simulink model "lab8_3and4"  (R2018b)
settings: Solver=FixedStepDiscrete  StartTime=0.0  StopTime=1000000  FixedStep=1  RelTol=1e-3
libraries: hdlsllib x4, simulink x2
settings Model: Creator=mllax8  LastModifiedBy=mllax8

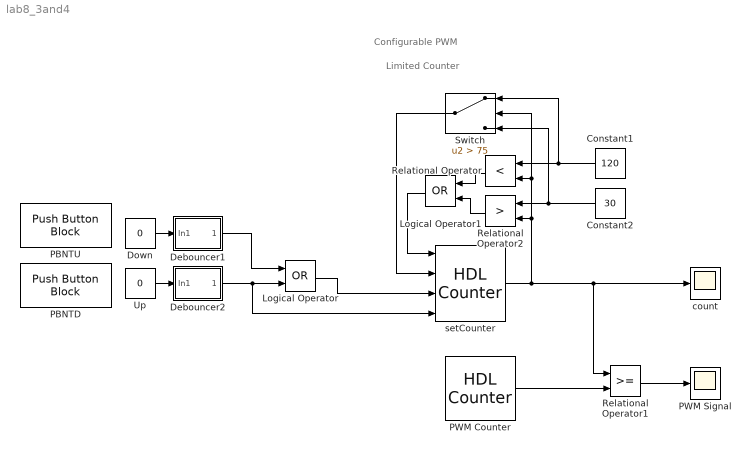
== system lab8_3and4 ==
  note: Configurable PWM
  note: Limited Counter
  Constant1 : Constant  Value=120  SampleTime=1
  Constant2 : Constant  Value=30  SampleTime=1
  Debouncer1 : Subsystem
  Debouncer2 : Subsystem
  Down : Constant  Value=0
  Logical Operator : Logic  Operator=OR  AllPortsSameDT=off  OutDataTypeStr=boolean
  Logical Operator1 : Logic  Operator=OR  AllPortsSameDT=off  OutDataTypeStr=boolean
  PBNTD : PushButtonBlock  WebBlockId=8
  PBNTU : PushButtonBlock  WebBlockId=9
  "PWM Counter " : hdlsllib/Sources/HDL Counter  CountType=Count limited  CountInit=0  CountStep=1  CountMax=1000  CountFromType=Initial value  CountFrom=0  CountResetPort=off  CountLoadPort=off  CountEnbPort=off  CountDirPort=off  CountDataType=Unsigned  CountWordLen=18  CountFracLen=0  CountSampTime=1
      settings: SourceProductBaseCode=HD
  PWM Signal : Scope
  Relational Operator : RelationalOperator  Operator=<  OutDataTypeStr=boolean  RndMeth=Simplest
  Relational Operator1 : RelationalOperator  OutDataTypeStr=boolean  RndMeth=Simplest
  Relational Operator2 : RelationalOperator  Operator=>  OutDataTypeStr=boolean  RndMeth=Simplest
  Switch : Switch  Criteria=u2 > Threshold  Threshold=75
  Up : Constant  Value=0
  count : Scope
  setCounter : hdlsllib/Sources/HDL Counter  CountType=Free running  CountInit=75  CountStep=6  CountMax=120  CountFromType=Initial value  CountFrom=75  CountResetPort=off  CountLoadPort=on  CountEnbPort=on  CountDirPort=on  CountDataType=Unsigned  CountWordLen=8  CountFracLen=0  CountSampTime=1
      settings: SourceProductBaseCode=HD
  wires:
  Down/1 -> Debouncer1/1(In1)
  Up/1 -> Debouncer2/1(In1)
  Debouncer1/1(Out1) -> Logical Operator/1
  Relational Operator1/1 -> PWM Signal/1
  Constant1/1 -> Switch/1, Relational Operator/1
  Constant2/1 -> Switch/3, Relational Operator2/1
  Logical Operator/1 -> setCounter/3
  Switch/1 -> setCounter/2
  Logical Operator1/1 -> setCounter/1
  setCounter/1 -> count/1, Relational Operator1/1, Switch/2, Relational Operator/2, Relational Operator2/2
  "PWM Counter "/1 -> Relational Operator1/2
  Relational Operator2/1 -> Logical Operator1/2
  Relational Operator/1 -> Logical Operator1/1
  Debouncer2/1(Out1) -> setCounter/4, Logical Operator/2

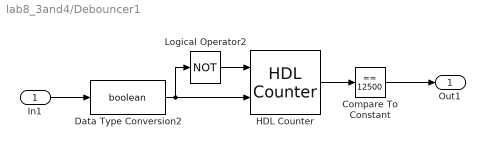
== system lab8_3and4/Debouncer1 ==
  In1 : Inport
  Compare To Constant : simulink/Logic and Bit Operations/Compare To Constant  relop===  const=12500  OutDataTypeStr=boolean
  Data Type Conversion2 : DataTypeConversion  OutDataTypeStr=boolean
  "HDL Counter " : hdlsllib/Sources/HDL Counter  CountType=Count limited  CountInit=0  CountStep=1  CountMax=50000  CountFromType=Initial value  CountFrom=0  CountResetPort=on  CountLoadPort=off  CountEnbPort=on  CountDirPort=off  CountDataType=Unsigned  CountWordLen=18  CountFracLen=0  CountSampTime=1
      settings: SourceProductBaseCode=HD
  Logical Operator2 : Logic  Operator=NOT  AllPortsSameDT=off  OutDataTypeStr=boolean
  Out1 : Outport
  wires:
  "HDL Counter "/1 -> Compare To Constant/1
  In1/1 -> Data Type Conversion2/1
  Logical Operator2/1 -> "HDL Counter "/1
  Compare To Constant/1 -> Out1/1
  Data Type Conversion2/1 -> "HDL Counter "/2, Logical Operator2/1

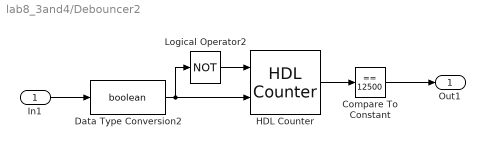
== system lab8_3and4/Debouncer2 ==
  In1 : Inport
  Compare To Constant : simulink/Logic and Bit Operations/Compare To Constant  relop===  const=12500  OutDataTypeStr=boolean
  Data Type Conversion2 : DataTypeConversion  OutDataTypeStr=boolean
  "HDL Counter " : hdlsllib/Sources/HDL Counter  CountType=Count limited  CountInit=0  CountStep=1  CountMax=50000  CountFromType=Initial value  CountFrom=0  CountResetPort=on  CountLoadPort=off  CountEnbPort=on  CountDirPort=off  CountDataType=Unsigned  CountWordLen=18  CountFracLen=0  CountSampTime=1
      settings: SourceProductBaseCode=HD
  Logical Operator2 : Logic  Operator=NOT  AllPortsSameDT=off  OutDataTypeStr=boolean
  Out1 : Outport
  wires:
  "HDL Counter "/1 -> Compare To Constant/1
  In1/1 -> Data Type Conversion2/1
  Logical Operator2/1 -> "HDL Counter "/1
  Compare To Constant/1 -> Out1/1
  Data Type Conversion2/1 -> "HDL Counter "/2, Logical Operator2/1
